simulink subsystem "S2"  (R2024b)
settings: Solver=VariableStepAuto  StartTime=0.0  StopTime=10.0  RelTol=1e-3
undefined symbols (not defined in the file): C, CC, DPL1ph, h, Half, Ll, nb_cell, numberOfCell, P_AC, Rdc, ResistanceM, Roff, Ron, Rt4, SampleTime, simetran, Ts, Zm
libraries: fl_lib x39, nesl_utility x33, ee_lib x20, simulink x6
(part 2 of 2)

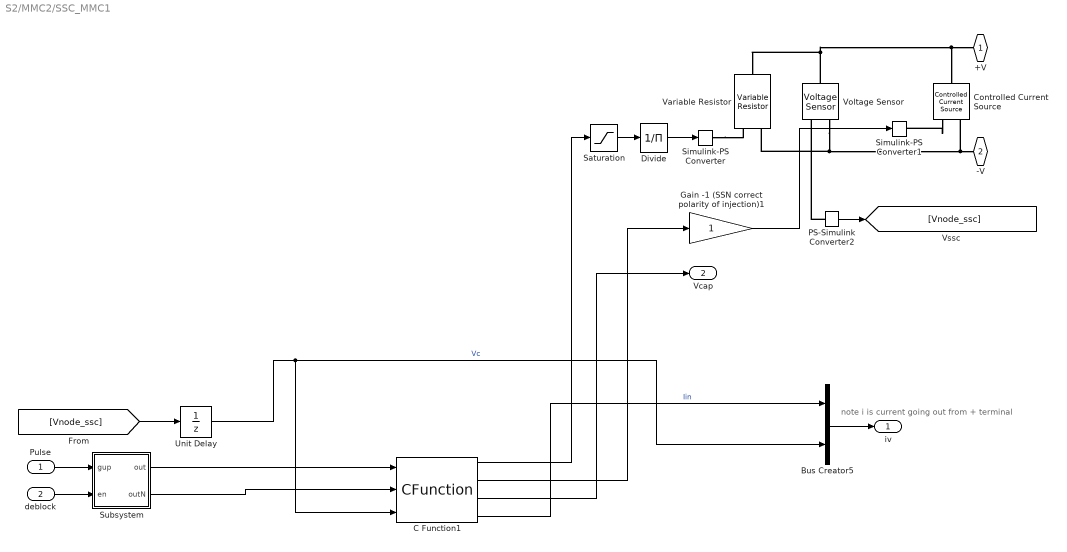
== system S2/MMC2/SSC_MMC1 ==
  note: note i is current going out from + terminal
  Pulse : Inport
  deblock : Inport  Port=2
  Bus Creator5 : BusCreator  Inputs=2
  C Function1 : CFunction  OutputCode=|  StartCode=state = initialValue;  InitializeConditionsCode=|  CodegenOutputCode=|  CodegenStartCode=state = initialValue;  CodegenInitializeConditionsCode=|  SampleTime=SampleTime  CustomCodeSettingLocation=ModelConfigurationParameters  initialValue=0  Ad=Ad  Bd2=Bd2  C=C  nbc=nbc  Z=Z  SampleTime=-1
      OutputCode=|
      | {
      | 
      | int ssx;
      | double Vcapasum, Ymmc, Zmmc, Vhist, Vterm;
      | double I;
      | 
      | Vcapasum=0;
      | I=(Vnodal- state_keep[0])* state_keep[1];  
      | 
      |     for (int k=0;k<nbc;k++){ //  % scan of cells to complete state-space iteration
      |         Vcap[k]=x_keep[k]+Bd2keep[k]*I;
      |         if (*(g_lower+k)<0.5) Vcapasum+=Vcap[k]; // sum all non-shorted capacitor voltages
      |     }
      | 
      | 
      |     Vhist=0;  // reset Vhist
      |     Zmmc=0;  // reset
      |     Vterm=  Vnodal;
      | 
      | 
      |     // we calculate the cells conduction states from the gate values.
      |     for (int k=0;k<nbc;k++){
      |         // ss=2-> lower IGBT/diode ON
      |         // ss=1-> upper IGBT/diode ON  //attention!!!!
      |         // ss=0-> hi-Z
      |         ssx=(int)gate[k];
      |         if (*(g_lower+k)>0.5) ssx=2;
      |         else if (*(g_upper+k)>0.5) ssx=1;
      |         else {
      |             if  (Vterm<0)  ssx=2;
      |             else if( Vterm>Vcapasum) ssx=1;
      |             else  ssx=0;
      |         }
      | 
      |         x_keep[k]=Ad[ssx]*Vcap[k];  //+Bd1[ssx]*I;    Bd1=0 avec backward Euler                                                          // note: with BE Bd1=0
      |         Vhist+=(C[ssx]*x_keep[k]);    //V_hist =V_hist + C(k)*state_tmp(k);  % compute Thevenin voltage
      | 
      |         Zmmc+=Z[ssx];  // Z = sum(C'.*Bd2 + D);  Y=inv(Z)
      | 
      |         Bd2keep[k]=Bd2[ssx];
      |         gate[k]=ssx;
      |         *(Vcap_out+k)=Vcap[k];
      |         }
      | 
      | 
      |     Ymmc=1/Zmmc;    // admittance= inverse of the sum of cell impedance
      |     Ihist=Vhist*Ymmc;  // history source
      | 
      |     state_keep[0]=Vhist;
      | 
      |     Y=Ymmc;
      | 
      |     state_keep[1]=Ymmc;
      | 
      |     Immc=0.0-I;
      | 
      | }
      InitializeConditionsCode=|
      | for (int i=0; i<nbc ;i++){
      |     x_keep[i]=0;
      |     Bd2keep[i]*0;
      |     Vc_state[i]=0;
      |     gate[i]=0;
      |     Vcap[i]=0;
      |     }
      |     
      |     state=0;
      |     state_keep[0]=0;
      |     state_keep[1]=0;
      CodegenOutputCode=|
      | {
      | 
      | int ssx;
      | double Vcapasum, Ymmc, Zmmc, Vhist, Vterm;
      | double I;
      | 
      | Vcapasum=0;
      | I=(Vnodal- state_keep[0])* state_keep[1];  
      | 
      |     for (int k=0;k<nbc;k++){ //  % scan of cells to complete state-space iteration
      |         Vcap[k]=x_keep[k]+Bd2keep[k]*I;
      |         if (*(g_lower+k)<0.5) Vcapasum+=Vcap[k]; // sum all non-shorted capacitor voltages
      |     }
      | 
      | 
      |     Vhist=0;  // reset Vhist
      |     Zmmc=0;  // reset
      |     Vterm=  Vnodal;
      | 
      | 
      |     // we calculate the cells conduction states from the gate values.
      |     for (int k=0;k<nbc;k++){
      |         // ss=2-> lower IGBT/diode ON
      |         // ss=1-> upper IGBT/diode ON  //attention!!!!
      |         // ss=0-> hi-Z
      |         ssx=(int)gate[k];
      |         if (*(g_lower+k)>0.5) ssx=2;
      |         else if (*(g_upper+k)>0.5) ssx=1;
      |         else {
      |             if  (Vterm<0)  ssx=2;
      |             else if( Vterm>Vcapasum) ssx=1;
      |             else  ssx=0;
      |         }
      | 
      |         x_keep[k]=Ad[ssx]*Vcap[k];  //+Bd1[ssx]*I;    Bd1=0 avec backward Euler                                                          // note: with BE Bd1=0
      |         Vhist+=(C[ssx]*x_keep[k]);    //V_hist =V_hist + C(k)*state_tmp(k);  % compute Thevenin voltage
      | 
      |         Zmmc+=Z[ssx];  // Z = sum(C'.*Bd2 + D);  Y=inv(Z)
      | 
      |         Bd2keep[k]=Bd2[ssx];
      |         gate[k]=ssx;
      |         *(Vcap_out+k)=Vcap[k];
      |         }
      | 
      | 
      |     Ymmc=1/Zmmc;    // admittance= inverse of the sum of cell impedance
      |     Ihist=Vhist*Ymmc;  // history source
      | 
      |     state_keep[0]=Vhist;
      | 
      |     Y=Ymmc;
      | 
      |     state_keep[1]=Ymmc;
      | 
      |     Immc=0.0-I;
      | 
      | }
      CodegenInitializeConditionsCode=|
      | for (int i=0; i<nbc ;i++){
      |     x_keep[i]=0;
      |     Bd2keep[i]*0;
      |     Vc_state[i]=0;
      |     gate[i]=0;
      |     Vcap[i]=0;
      |     }
      |     
      |     state=0;
      |     state_keep[0]=0;
      |     state_keep[1]=0;
  Controlled Current Source : fl_lib/Electrical/Electrical Sources/Controlled Current Source
  Divide : Product  Inputs=/
  Gain -1 (SSN correct polarity of injection)1 : Gain
  PS-Simulink Converter2 : nesl_utility/PS-Simulink Converter  PhysicalDomain=network_engine_domain  SubClassName=ps_output  LeftPortType=input  RightPortType=output  PseudoPeriodic=off  Frequencies=[]  VectorFormat=inherit  Unit=inherit  AffineConversion=off
  Saturation : Saturate  UpperLimit=1e9  LowerLimit=0
  Simulink-PS Converter : nesl_utility/Simulink-PS Converter  PhysicalDomain=network_engine_domain  SubClassName=ps_input  LeftPortType=input  RightPortType=output  PseudoPeriodic=off  Frequencies=[]  NoiseDistribution=none  NoiseParameters=[]  Unit=1  AffineConversion=off  FilteringAndDerivatives=provide  SimscapeFilterOrder=1  InputFilterTimeConstant=0.001  UdotUserProvided=0
  Simulink-PS Converter1 : nesl_utility/Simulink-PS Converter  PhysicalDomain=network_engine_domain  SubClassName=ps_input  LeftPortType=input  RightPortType=output  PseudoPeriodic=off  Frequencies=[]  NoiseDistribution=none  NoiseParameters=[]  Unit=1  AffineConversion=off  FilteringAndDerivatives=provide  SimscapeFilterOrder=1  InputFilterTimeConstant=0.001  UdotUserProvided=0
  Subsystem : Subsystem  mask(MMC pulsing){nbc=nbc}
      mask prompts: nbc "Number of Cells"
      mask init:
      | igbtorder=[];
      | for i=1:nbc
      |     igbtorder=[igbtorder i i+nbc];
      | end
      | igbtorder;
  Unit Delay : UnitDelay  SampleTime=Ts  HasFrameUpgradeWarning=on
  Variable Resistor : fl_lib/Electrical/Electrical Elements/Variable Resistor  Rmin=1e-8 Ohm  thermalEnable=false  thermal_mass=1 J/K  i_specify=off  i_priority=None  i=0 A  i_nominal_specify=off  i_nominal_value=1  i_nominal_unit=A  v_specify=off  v_priority=None  v=0 V  v_nominal_specify=off  v_nominal_value=1  v_nominal_unit=V  T_specify=off  T_priority=None  T=300 K  T_nominal_specify=off  T_nominal_value=1  T_nominal_unit=K
  Voltage Sensor : fl_lib/Electrical/Electrical Sensors/Voltage Sensor
  +V : PMIOPort  Side=Left
  -V : PMIOPort  Port=2  Side=Left
  iv : Outport  VectorParamsAs1DForOutWhenUnconnected=off
  Vcap : Outport  Port=2  VectorParamsAs1DForOutWhenUnconnected=off
  wires:
  C Function1/4 -> Bus Creator5/1  "Iin"
  C Function1/3 -> Vcap/1
  C Function1/2 -> Gain -1 (SSN correct polarity of injection)1/1
  C Function1/1 -> Saturation/1
  Unit Delay/1 -> Bus Creator5/2, C Function1/3  "Vc"
  Bus Creator5/1 -> iv/1
  Subsystem/1(out) -> C Function1/1
  Pulse/1 -> Subsystem/1(gup)
  Subsystem/2(outN) -> C Function1/2
  deblock/1 -> Subsystem/2(en)
  PS-Simulink Converter2/1 -> [Vnode_ssc]
  [Vnode_ssc] -> Unit Delay/1
  Gain -1 (SSN correct polarity of injection)1/1 -> Simulink-PS Converter1/1
  Divide/1 -> Simulink-PS Converter/1
  Saturation/1 -> Divide/1
  connections:
  Simulink-PS Converter/RConn1 -- Variable Resistor/LConn1
  Voltage Sensor/RConn2 -- Controlled Current Source/RConn2 -- -V/RConn1 -- Variable Resistor/LConn2
  Voltage Sensor/LConn1 -- Controlled Current Source/LConn1 -- +V/RConn1 -- Variable Resistor/RConn1
  PS-Simulink Converter2/LConn1 -- Voltage Sensor/RConn1
  Controlled Current Source/RConn1 -- Simulink-PS Converter1/RConn1

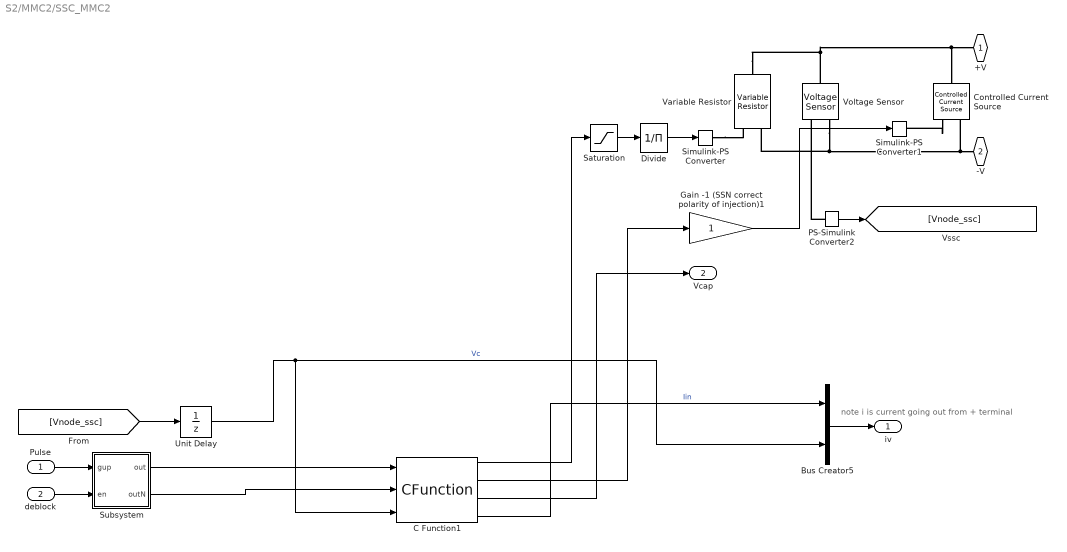
== system S2/MMC2/SSC_MMC2 ==
  note: note i is current going out from + terminal
  Pulse : Inport
  deblock : Inport  Port=2
  Bus Creator5 : BusCreator  Inputs=2
  C Function1 : CFunction  OutputCode=|  StartCode=state = initialValue;  InitializeConditionsCode=|  CodegenOutputCode=|  CodegenStartCode=state = initialValue;  CodegenInitializeConditionsCode=|  SampleTime=SampleTime  CustomCodeSettingLocation=ModelConfigurationParameters  initialValue=0  Ad=Ad  Bd2=Bd2  C=C  nbc=nbc  Z=Z  SampleTime=-1
      OutputCode=|
      | {
      | 
      | int ssx;
      | double Vcapasum, Ymmc, Zmmc, Vhist, Vterm;
      | double I;
      | 
      | Vcapasum=0;
      | I=(Vnodal- state_keep[0])* state_keep[1];  
      | 
      |     for (int k=0;k<nbc;k++){ //  % scan of cells to complete state-space iteration
      |         Vcap[k]=x_keep[k]+Bd2keep[k]*I;
      |         if (*(g_lower+k)<0.5) Vcapasum+=Vcap[k]; // sum all non-shorted capacitor voltages
      |     }
      | 
      | 
      |     Vhist=0;  // reset Vhist
      |     Zmmc=0;  // reset
      |     Vterm=  Vnodal;
      | 
      | 
      |     // we calculate the cells conduction states from the gate values.
      |     for (int k=0;k<nbc;k++){
      |         // ss=2-> lower IGBT/diode ON
      |         // ss=1-> upper IGBT/diode ON  //attention!!!!
      |         // ss=0-> hi-Z
      |         ssx=(int)gate[k];
      |         if (*(g_lower+k)>0.5) ssx=2;
      |         else if (*(g_upper+k)>0.5) ssx=1;
      |         else {
      |             if  (Vterm<0)  ssx=2;
      |             else if( Vterm>Vcapasum) ssx=1;
      |             else  ssx=0;
      |         }
      | 
      |         x_keep[k]=Ad[ssx]*Vcap[k];  //+Bd1[ssx]*I;    Bd1=0 avec backward Euler                                                          // note: with BE Bd1=0
      |         Vhist+=(C[ssx]*x_keep[k]);    //V_hist =V_hist + C(k)*state_tmp(k);  % compute Thevenin voltage
      | 
      |         Zmmc+=Z[ssx];  // Z = sum(C'.*Bd2 + D);  Y=inv(Z)
      | 
      |         Bd2keep[k]=Bd2[ssx];
      |         gate[k]=ssx;
      |         *(Vcap_out+k)=Vcap[k];
      |         }
      | 
      | 
      |     Ymmc=1/Zmmc;    // admittance= inverse of the sum of cell impedance
      |     Ihist=Vhist*Ymmc;  // history source
      | 
      |     state_keep[0]=Vhist;
      | 
      |     Y=Ymmc;
      | 
      |     state_keep[1]=Ymmc;
      | 
      |     Immc=0.0-I;
      | 
      | }
      InitializeConditionsCode=|
      | for (int i=0; i<nbc ;i++){
      |     x_keep[i]=0;
      |     Bd2keep[i]*0;
      |     Vc_state[i]=0;
      |     gate[i]=0;
      |     Vcap[i]=0;
      |     }
      |     
      |     state=0;
      |     state_keep[0]=0;
      |     state_keep[1]=0;
      CodegenOutputCode=|
      | {
      | 
      | int ssx;
      | double Vcapasum, Ymmc, Zmmc, Vhist, Vterm;
      | double I;
      | 
      | Vcapasum=0;
      | I=(Vnodal- state_keep[0])* state_keep[1];  
      | 
      |     for (int k=0;k<nbc;k++){ //  % scan of cells to complete state-space iteration
      |         Vcap[k]=x_keep[k]+Bd2keep[k]*I;
      |         if (*(g_lower+k)<0.5) Vcapasum+=Vcap[k]; // sum all non-shorted capacitor voltages
      |     }
      | 
      | 
      |     Vhist=0;  // reset Vhist
      |     Zmmc=0;  // reset
      |     Vterm=  Vnodal;
      | 
      | 
      |     // we calculate the cells conduction states from the gate values.
      |     for (int k=0;k<nbc;k++){
      |         // ss=2-> lower IGBT/diode ON
      |         // ss=1-> upper IGBT/diode ON  //attention!!!!
      |         // ss=0-> hi-Z
      |         ssx=(int)gate[k];
      |         if (*(g_lower+k)>0.5) ssx=2;
      |         else if (*(g_upper+k)>0.5) ssx=1;
      |         else {
      |             if  (Vterm<0)  ssx=2;
      |             else if( Vterm>Vcapasum) ssx=1;
      |             else  ssx=0;
      |         }
      | 
      |         x_keep[k]=Ad[ssx]*Vcap[k];  //+Bd1[ssx]*I;    Bd1=0 avec backward Euler                                                          // note: with BE Bd1=0
      |         Vhist+=(C[ssx]*x_keep[k]);    //V_hist =V_hist + C(k)*state_tmp(k);  % compute Thevenin voltage
      | 
      |         Zmmc+=Z[ssx];  // Z = sum(C'.*Bd2 + D);  Y=inv(Z)
      | 
      |         Bd2keep[k]=Bd2[ssx];
      |         gate[k]=ssx;
      |         *(Vcap_out+k)=Vcap[k];
      |         }
      | 
      | 
      |     Ymmc=1/Zmmc;    // admittance= inverse of the sum of cell impedance
      |     Ihist=Vhist*Ymmc;  // history source
      | 
      |     state_keep[0]=Vhist;
      | 
      |     Y=Ymmc;
      | 
      |     state_keep[1]=Ymmc;
      | 
      |     Immc=0.0-I;
      | 
      | }
      CodegenInitializeConditionsCode=|
      | for (int i=0; i<nbc ;i++){
      |     x_keep[i]=0;
      |     Bd2keep[i]*0;
      |     Vc_state[i]=0;
      |     gate[i]=0;
      |     Vcap[i]=0;
      |     }
      |     
      |     state=0;
      |     state_keep[0]=0;
      |     state_keep[1]=0;
  Controlled Current Source : fl_lib/Electrical/Electrical Sources/Controlled Current Source
  Divide : Product  Inputs=/
  Gain -1 (SSN correct polarity of injection)1 : Gain
  PS-Simulink Converter2 : nesl_utility/PS-Simulink Converter  PhysicalDomain=network_engine_domain  SubClassName=ps_output  LeftPortType=input  RightPortType=output  PseudoPeriodic=off  Frequencies=[]  VectorFormat=inherit  Unit=inherit  AffineConversion=off
  Saturation : Saturate  UpperLimit=1e9  LowerLimit=0
  Simulink-PS Converter : nesl_utility/Simulink-PS Converter  PhysicalDomain=network_engine_domain  SubClassName=ps_input  LeftPortType=input  RightPortType=output  PseudoPeriodic=off  Frequencies=[]  NoiseDistribution=none  NoiseParameters=[]  Unit=1  AffineConversion=off  FilteringAndDerivatives=provide  SimscapeFilterOrder=1  InputFilterTimeConstant=0.001  UdotUserProvided=0
  Simulink-PS Converter1 : nesl_utility/Simulink-PS Converter  PhysicalDomain=network_engine_domain  SubClassName=ps_input  LeftPortType=input  RightPortType=output  PseudoPeriodic=off  Frequencies=[]  NoiseDistribution=none  NoiseParameters=[]  Unit=1  AffineConversion=off  FilteringAndDerivatives=provide  SimscapeFilterOrder=1  InputFilterTimeConstant=0.001  UdotUserProvided=0
  Subsystem : Subsystem  mask(MMC pulsing){nbc=nbc}
      mask prompts: nbc "Number of Cells"
      mask init:
      | igbtorder=[];
      | for i=1:nbc
      |     igbtorder=[igbtorder i i+nbc];
      | end
      | igbtorder;
  Unit Delay : UnitDelay  SampleTime=Ts  HasFrameUpgradeWarning=on
  Variable Resistor : fl_lib/Electrical/Electrical Elements/Variable Resistor  Rmin=1e-8 Ohm  thermalEnable=false  thermal_mass=1 J/K  i_specify=off  i_priority=None  i=0 A  i_nominal_specify=off  i_nominal_value=1  i_nominal_unit=A  v_specify=off  v_priority=None  v=0 V  v_nominal_specify=off  v_nominal_value=1  v_nominal_unit=V  T_specify=off  T_priority=None  T=300 K  T_nominal_specify=off  T_nominal_value=1  T_nominal_unit=K
  Voltage Sensor : fl_lib/Electrical/Electrical Sensors/Voltage Sensor
  +V : PMIOPort  Side=Left
  -V : PMIOPort  Port=2  Side=Left
  iv : Outport  VectorParamsAs1DForOutWhenUnconnected=off
  Vcap : Outport  Port=2  VectorParamsAs1DForOutWhenUnconnected=off
  wires:
  Saturation/1 -> Divide/1
  Divide/1 -> Simulink-PS Converter/1
  Gain -1 (SSN correct polarity of injection)1/1 -> Simulink-PS Converter1/1
  [Vnode_ssc] -> Unit Delay/1
  PS-Simulink Converter2/1 -> [Vnode_ssc]
  deblock/1 -> Subsystem/2(en)
  Subsystem/2(outN) -> C Function1/2
  Pulse/1 -> Subsystem/1(gup)
  Subsystem/1(out) -> C Function1/1
  Bus Creator5/1 -> iv/1
  Unit Delay/1 -> C Function1/3, Bus Creator5/2  "Vc"
  C Function1/1 -> Saturation/1
  C Function1/2 -> Gain -1 (SSN correct polarity of injection)1/1
  C Function1/3 -> Vcap/1
  C Function1/4 -> Bus Creator5/1  "Iin"
  connections:
  Controlled Current Source/RConn1 -- Simulink-PS Converter1/RConn1
  PS-Simulink Converter2/LConn1 -- Voltage Sensor/RConn1
  Variable Resistor/RConn1 -- +V/RConn1 -- Controlled Current Source/LConn1 -- Voltage Sensor/LConn1
  Variable Resistor/LConn2 -- -V/RConn1 -- Controlled Current Source/RConn2 -- Voltage Sensor/RConn2
  Simulink-PS Converter/RConn1 -- Variable Resistor/LConn1

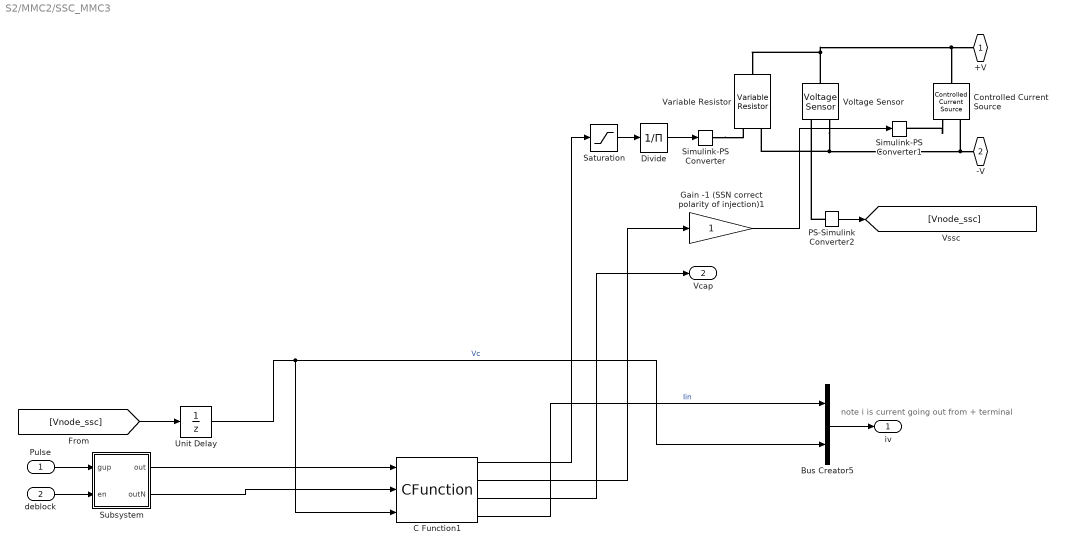
== system S2/MMC2/SSC_MMC3 ==
  note: note i is current going out from + terminal
  Pulse : Inport
  deblock : Inport  Port=2
  Bus Creator5 : BusCreator  Inputs=2
  C Function1 : CFunction  OutputCode=|  StartCode=state = initialValue;  InitializeConditionsCode=|  CodegenOutputCode=|  CodegenStartCode=state = initialValue;  CodegenInitializeConditionsCode=|  SampleTime=SampleTime  CustomCodeSettingLocation=ModelConfigurationParameters  initialValue=0  Ad=Ad  Bd2=Bd2  C=C  nbc=nbc  Z=Z  SampleTime=-1
      OutputCode=|
      | {
      | 
      | int ssx;
      | double Vcapasum, Ymmc, Zmmc, Vhist, Vterm;
      | double I;
      | 
      | Vcapasum=0;
      | I=(Vnodal- state_keep[0])* state_keep[1];  
      | 
      |     for (int k=0;k<nbc;k++){ //  % scan of cells to complete state-space iteration
      |         Vcap[k]=x_keep[k]+Bd2keep[k]*I;
      |         if (*(g_lower+k)<0.5) Vcapasum+=Vcap[k]; // sum all non-shorted capacitor voltages
      |     }
      | 
      | 
      |     Vhist=0;  // reset Vhist
      |     Zmmc=0;  // reset
      |     Vterm=  Vnodal;
      | 
      | 
      |     // we calculate the cells conduction states from the gate values.
      |     for (int k=0;k<nbc;k++){
      |         // ss=2-> lower IGBT/diode ON
      |         // ss=1-> upper IGBT/diode ON  //attention!!!!
      |         // ss=0-> hi-Z
      |         ssx=(int)gate[k];
      |         if (*(g_lower+k)>0.5) ssx=2;
      |         else if (*(g_upper+k)>0.5) ssx=1;
      |         else {
      |             if  (Vterm<0)  ssx=2;
      |             else if( Vterm>Vcapasum) ssx=1;
      |             else  ssx=0;
      |         }
      | 
      |         x_keep[k]=Ad[ssx]*Vcap[k];  //+Bd1[ssx]*I;    Bd1=0 avec backward Euler                                                          // note: with BE Bd1=0
      |         Vhist+=(C[ssx]*x_keep[k]);    //V_hist =V_hist + C(k)*state_tmp(k);  % compute Thevenin voltage
      | 
      |         Zmmc+=Z[ssx];  // Z = sum(C'.*Bd2 + D);  Y=inv(Z)
      | 
      |         Bd2keep[k]=Bd2[ssx];
      |         gate[k]=ssx;
      |         *(Vcap_out+k)=Vcap[k];
      |         }
      | 
      | 
      |     Ymmc=1/Zmmc;    // admittance= inverse of the sum of cell impedance
      |     Ihist=Vhist*Ymmc;  // history source
      | 
      |     state_keep[0]=Vhist;
      | 
      |     Y=Ymmc;
      | 
      |     state_keep[1]=Ymmc;
      | 
      |     Immc=0.0-I;
      | 
      | }
      InitializeConditionsCode=|
      | for (int i=0; i<nbc ;i++){
      |     x_keep[i]=0;
      |     Bd2keep[i]*0;
      |     Vc_state[i]=0;
      |     gate[i]=0;
      |     Vcap[i]=0;
      |     }
      |     
      |     state=0;
      |     state_keep[0]=0;
      |     state_keep[1]=0;
      CodegenOutputCode=|
      | {
      | 
      | int ssx;
      | double Vcapasum, Ymmc, Zmmc, Vhist, Vterm;
      | double I;
      | 
      | Vcapasum=0;
      | I=(Vnodal- state_keep[0])* state_keep[1];  
      | 
      |     for (int k=0;k<nbc;k++){ //  % scan of cells to complete state-space iteration
      |         Vcap[k]=x_keep[k]+Bd2keep[k]*I;
      |         if (*(g_lower+k)<0.5) Vcapasum+=Vcap[k]; // sum all non-shorted capacitor voltages
      |     }
      | 
      | 
      |     Vhist=0;  // reset Vhist
      |     Zmmc=0;  // reset
      |     Vterm=  Vnodal;
      | 
      | 
      |     // we calculate the cells conduction states from the gate values.
      |     for (int k=0;k<nbc;k++){
      |         // ss=2-> lower IGBT/diode ON
      |         // ss=1-> upper IGBT/diode ON  //attention!!!!
      |         // ss=0-> hi-Z
      |         ssx=(int)gate[k];
      |         if (*(g_lower+k)>0.5) ssx=2;
      |         else if (*(g_upper+k)>0.5) ssx=1;
      |         else {
      |             if  (Vterm<0)  ssx=2;
      |             else if( Vterm>Vcapasum) ssx=1;
      |             else  ssx=0;
      |         }
      | 
      |         x_keep[k]=Ad[ssx]*Vcap[k];  //+Bd1[ssx]*I;    Bd1=0 avec backward Euler                                                          // note: with BE Bd1=0
      |         Vhist+=(C[ssx]*x_keep[k]);    //V_hist =V_hist + C(k)*state_tmp(k);  % compute Thevenin voltage
      | 
      |         Zmmc+=Z[ssx];  // Z = sum(C'.*Bd2 + D);  Y=inv(Z)
      | 
      |         Bd2keep[k]=Bd2[ssx];
      |         gate[k]=ssx;
      |         *(Vcap_out+k)=Vcap[k];
      |         }
      | 
      | 
      |     Ymmc=1/Zmmc;    // admittance= inverse of the sum of cell impedance
      |     Ihist=Vhist*Ymmc;  // history source
      | 
      |     state_keep[0]=Vhist;
      | 
      |     Y=Ymmc;
      | 
      |     state_keep[1]=Ymmc;
      | 
      |     Immc=0.0-I;
      | 
      | }
      CodegenInitializeConditionsCode=|
      | for (int i=0; i<nbc ;i++){
      |     x_keep[i]=0;
      |     Bd2keep[i]*0;
      |     Vc_state[i]=0;
      |     gate[i]=0;
      |     Vcap[i]=0;
      |     }
      |     
      |     state=0;
      |     state_keep[0]=0;
      |     state_keep[1]=0;
  Controlled Current Source : fl_lib/Electrical/Electrical Sources/Controlled Current Source
  Divide : Product  Inputs=/
  Gain -1 (SSN correct polarity of injection)1 : Gain
  PS-Simulink Converter2 : nesl_utility/PS-Simulink Converter  PhysicalDomain=network_engine_domain  SubClassName=ps_output  LeftPortType=input  RightPortType=output  PseudoPeriodic=off  Frequencies=[]  VectorFormat=inherit  Unit=inherit  AffineConversion=off
  Saturation : Saturate  UpperLimit=1e9  LowerLimit=0
  Simulink-PS Converter : nesl_utility/Simulink-PS Converter  PhysicalDomain=network_engine_domain  SubClassName=ps_input  LeftPortType=input  RightPortType=output  PseudoPeriodic=off  Frequencies=[]  NoiseDistribution=none  NoiseParameters=[]  Unit=1  AffineConversion=off  FilteringAndDerivatives=provide  SimscapeFilterOrder=1  InputFilterTimeConstant=0.001  UdotUserProvided=0
  Simulink-PS Converter1 : nesl_utility/Simulink-PS Converter  PhysicalDomain=network_engine_domain  SubClassName=ps_input  LeftPortType=input  RightPortType=output  PseudoPeriodic=off  Frequencies=[]  NoiseDistribution=none  NoiseParameters=[]  Unit=1  AffineConversion=off  FilteringAndDerivatives=provide  SimscapeFilterOrder=1  InputFilterTimeConstant=0.001  UdotUserProvided=0
  Subsystem : Subsystem  mask(MMC pulsing){nbc=nbc}
      mask prompts: nbc "Number of Cells"
      mask init:
      | igbtorder=[];
      | for i=1:nbc
      |     igbtorder=[igbtorder i i+nbc];
      | end
      | igbtorder;
  Unit Delay : UnitDelay  SampleTime=Ts  HasFrameUpgradeWarning=on
  Variable Resistor : fl_lib/Electrical/Electrical Elements/Variable Resistor  Rmin=1e-8 Ohm  thermalEnable=false  thermal_mass=1 J/K  i_specify=off  i_priority=None  i=0 A  i_nominal_specify=off  i_nominal_value=1  i_nominal_unit=A  v_specify=off  v_priority=None  v=0 V  v_nominal_specify=off  v_nominal_value=1  v_nominal_unit=V  T_specify=off  T_priority=None  T=300 K  T_nominal_specify=off  T_nominal_value=1  T_nominal_unit=K
  Voltage Sensor : fl_lib/Electrical/Electrical Sensors/Voltage Sensor
  +V : PMIOPort  Side=Left
  -V : PMIOPort  Port=2  Side=Left
  iv : Outport  VectorParamsAs1DForOutWhenUnconnected=off
  Vcap : Outport  Port=2  VectorParamsAs1DForOutWhenUnconnected=off
  wires:
  C Function1/4 -> Bus Creator5/1  "Iin"
  C Function1/3 -> Vcap/1
  C Function1/2 -> Gain -1 (SSN correct polarity of injection)1/1
  C Function1/1 -> Saturation/1
  Unit Delay/1 -> Bus Creator5/2, C Function1/3  "Vc"
  Bus Creator5/1 -> iv/1
  Subsystem/1(out) -> C Function1/1
  Pulse/1 -> Subsystem/1(gup)
  Subsystem/2(outN) -> C Function1/2
  deblock/1 -> Subsystem/2(en)
  PS-Simulink Converter2/1 -> [Vnode_ssc]
  [Vnode_ssc] -> Unit Delay/1
  Gain -1 (SSN correct polarity of injection)1/1 -> Simulink-PS Converter1/1
  Divide/1 -> Simulink-PS Converter/1
  Saturation/1 -> Divide/1
  connections:
  Simulink-PS Converter/RConn1 -- Variable Resistor/LConn1
  Voltage Sensor/RConn2 -- Controlled Current Source/RConn2 -- -V/RConn1 -- Variable Resistor/LConn2
  Voltage Sensor/LConn1 -- Controlled Current Source/LConn1 -- +V/RConn1 -- Variable Resistor/RConn1
  PS-Simulink Converter2/LConn1 -- Voltage Sensor/RConn1
  Controlled Current Source/RConn1 -- Simulink-PS Converter1/RConn1

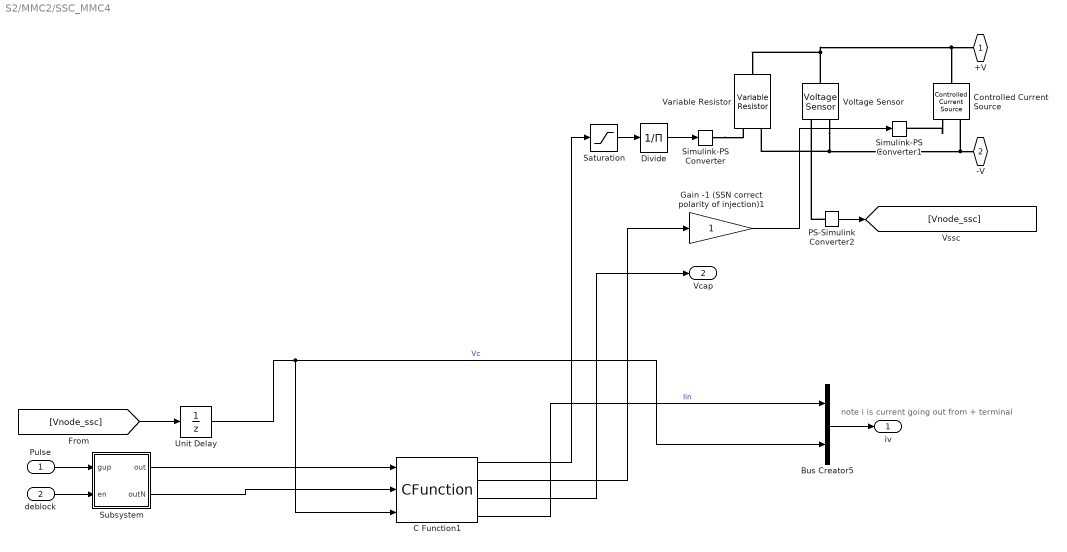
== system S2/MMC2/SSC_MMC4 ==
  note: note i is current going out from + terminal
  Pulse : Inport
  deblock : Inport  Port=2
  Bus Creator5 : BusCreator  Inputs=2
  C Function1 : CFunction  OutputCode=|  StartCode=state = initialValue;  InitializeConditionsCode=|  CodegenOutputCode=|  CodegenStartCode=state = initialValue;  CodegenInitializeConditionsCode=|  SampleTime=SampleTime  CustomCodeSettingLocation=ModelConfigurationParameters  initialValue=0  Ad=Ad  Bd2=Bd2  C=C  nbc=nbc  Z=Z  SampleTime=-1
      OutputCode=|
      | {
      | 
      | int ssx;
      | double Vcapasum, Ymmc, Zmmc, Vhist, Vterm;
      | double I;
      | 
      | Vcapasum=0;
      | I=(Vnodal- state_keep[0])* state_keep[1];  
      | 
      |     for (int k=0;k<nbc;k++){ //  % scan of cells to complete state-space iteration
      |         Vcap[k]=x_keep[k]+Bd2keep[k]*I;
      |         if (*(g_lower+k)<0.5) Vcapasum+=Vcap[k]; // sum all non-shorted capacitor voltages
      |     }
      | 
      | 
      |     Vhist=0;  // reset Vhist
      |     Zmmc=0;  // reset
      |     Vterm=  Vnodal;
      | 
      | 
      |     // we calculate the cells conduction states from the gate values.
      |     for (int k=0;k<nbc;k++){
      |         // ss=2-> lower IGBT/diode ON
      |         // ss=1-> upper IGBT/diode ON  //attention!!!!
      |         // ss=0-> hi-Z
      |         ssx=(int)gate[k];
      |         if (*(g_lower+k)>0.5) ssx=2;
      |         else if (*(g_upper+k)>0.5) ssx=1;
      |         else {
      |             if  (Vterm<0)  ssx=2;
      |             else if( Vterm>Vcapasum) ssx=1;
      |             else  ssx=0;
      |         }
      | 
      |         x_keep[k]=Ad[ssx]*Vcap[k];  //+Bd1[ssx]*I;    Bd1=0 avec backward Euler                                                          // note: with BE Bd1=0
      |         Vhist+=(C[ssx]*x_keep[k]);    //V_hist =V_hist + C(k)*state_tmp(k);  % compute Thevenin voltage
      | 
      |         Zmmc+=Z[ssx];  // Z = sum(C'.*Bd2 + D);  Y=inv(Z)
      | 
      |         Bd2keep[k]=Bd2[ssx];
      |         gate[k]=ssx;
      |         *(Vcap_out+k)=Vcap[k];
      |         }
      | 
      | 
      |     Ymmc=1/Zmmc;    // admittance= inverse of the sum of cell impedance
      |     Ihist=Vhist*Ymmc;  // history source
      | 
      |     state_keep[0]=Vhist;
      | 
      |     Y=Ymmc;
      | 
      |     state_keep[1]=Ymmc;
      | 
      |     Immc=0.0-I;
      | 
      | }
      InitializeConditionsCode=|
      | for (int i=0; i<nbc ;i++){
      |     x_keep[i]=0;
      |     Bd2keep[i]*0;
      |     Vc_state[i]=0;
      |     gate[i]=0;
      |     Vcap[i]=0;
      |     }
      |     
      |     state=0;
      |     state_keep[0]=0;
      |     state_keep[1]=0;
      CodegenOutputCode=|
      | {
      | 
      | int ssx;
      | double Vcapasum, Ymmc, Zmmc, Vhist, Vterm;
      | double I;
      | 
      | Vcapasum=0;
      | I=(Vnodal- state_keep[0])* state_keep[1];  
      | 
      |     for (int k=0;k<nbc;k++){ //  % scan of cells to complete state-space iteration
      |         Vcap[k]=x_keep[k]+Bd2keep[k]*I;
      |         if (*(g_lower+k)<0.5) Vcapasum+=Vcap[k]; // sum all non-shorted capacitor voltages
      |     }
      | 
      | 
      |     Vhist=0;  // reset Vhist
      |     Zmmc=0;  // reset
      |     Vterm=  Vnodal;
      | 
      | 
      |     // we calculate the cells conduction states from the gate values.
      |     for (int k=0;k<nbc;k++){
      |         // ss=2-> lower IGBT/diode ON
      |         // ss=1-> upper IGBT/diode ON  //attention!!!!
      |         // ss=0-> hi-Z
      |         ssx=(int)gate[k];
      |         if (*(g_lower+k)>0.5) ssx=2;
      |         else if (*(g_upper+k)>0.5) ssx=1;
      |         else {
      |             if  (Vterm<0)  ssx=2;
      |             else if( Vterm>Vcapasum) ssx=1;
      |             else  ssx=0;
      |         }
      | 
      |         x_keep[k]=Ad[ssx]*Vcap[k];  //+Bd1[ssx]*I;    Bd1=0 avec backward Euler                                                          // note: with BE Bd1=0
      |         Vhist+=(C[ssx]*x_keep[k]);    //V_hist =V_hist + C(k)*state_tmp(k);  % compute Thevenin voltage
      | 
      |         Zmmc+=Z[ssx];  // Z = sum(C'.*Bd2 + D);  Y=inv(Z)
      | 
      |         Bd2keep[k]=Bd2[ssx];
      |         gate[k]=ssx;
      |         *(Vcap_out+k)=Vcap[k];
      |         }
      | 
      | 
      |     Ymmc=1/Zmmc;    // admittance= inverse of the sum of cell impedance
      |     Ihist=Vhist*Ymmc;  // history source
      | 
      |     state_keep[0]=Vhist;
      | 
      |     Y=Ymmc;
      | 
      |     state_keep[1]=Ymmc;
      | 
      |     Immc=0.0-I;
      | 
      | }
      CodegenInitializeConditionsCode=|
      | for (int i=0; i<nbc ;i++){
      |     x_keep[i]=0;
      |     Bd2keep[i]*0;
      |     Vc_state[i]=0;
      |     gate[i]=0;
      |     Vcap[i]=0;
      |     }
      |     
      |     state=0;
      |     state_keep[0]=0;
      |     state_keep[1]=0;
  Controlled Current Source : fl_lib/Electrical/Electrical Sources/Controlled Current Source
  Divide : Product  Inputs=/
  Gain -1 (SSN correct polarity of injection)1 : Gain
  PS-Simulink Converter2 : nesl_utility/PS-Simulink Converter  PhysicalDomain=network_engine_domain  SubClassName=ps_output  LeftPortType=input  RightPortType=output  PseudoPeriodic=off  Frequencies=[]  VectorFormat=inherit  Unit=inherit  AffineConversion=off
  Saturation : Saturate  UpperLimit=1e9  LowerLimit=0
  Simulink-PS Converter : nesl_utility/Simulink-PS Converter  PhysicalDomain=network_engine_domain  SubClassName=ps_input  LeftPortType=input  RightPortType=output  PseudoPeriodic=off  Frequencies=[]  NoiseDistribution=none  NoiseParameters=[]  Unit=1  AffineConversion=off  FilteringAndDerivatives=provide  SimscapeFilterOrder=1  InputFilterTimeConstant=0.001  UdotUserProvided=0
  Simulink-PS Converter1 : nesl_utility/Simulink-PS Converter  PhysicalDomain=network_engine_domain  SubClassName=ps_input  LeftPortType=input  RightPortType=output  PseudoPeriodic=off  Frequencies=[]  NoiseDistribution=none  NoiseParameters=[]  Unit=1  AffineConversion=off  FilteringAndDerivatives=provide  SimscapeFilterOrder=1  InputFilterTimeConstant=0.001  UdotUserProvided=0
  Subsystem : Subsystem  mask(MMC pulsing){nbc=nbc}
      mask prompts: nbc "Number of Cells"
      mask init:
      | igbtorder=[];
      | for i=1:nbc
      |     igbtorder=[igbtorder i i+nbc];
      | end
      | igbtorder;
  Unit Delay : UnitDelay  SampleTime=Ts  HasFrameUpgradeWarning=on
  Variable Resistor : fl_lib/Electrical/Electrical Elements/Variable Resistor  Rmin=1e-8 Ohm  thermalEnable=false  thermal_mass=1 J/K  i_specify=off  i_priority=None  i=0 A  i_nominal_specify=off  i_nominal_value=1  i_nominal_unit=A  v_specify=off  v_priority=None  v=0 V  v_nominal_specify=off  v_nominal_value=1  v_nominal_unit=V  T_specify=off  T_priority=None  T=300 K  T_nominal_specify=off  T_nominal_value=1  T_nominal_unit=K
  Voltage Sensor : fl_lib/Electrical/Electrical Sensors/Voltage Sensor
  +V : PMIOPort  Side=Left
  -V : PMIOPort  Port=2  Side=Left
  iv : Outport  VectorParamsAs1DForOutWhenUnconnected=off
  Vcap : Outport  Port=2  VectorParamsAs1DForOutWhenUnconnected=off
  wires:
  C Function1/4 -> Bus Creator5/1  "Iin"
  C Function1/3 -> Vcap/1
  C Function1/2 -> Gain -1 (SSN correct polarity of injection)1/1
  C Function1/1 -> Saturation/1
  Unit Delay/1 -> Bus Creator5/2, C Function1/3  "Vc"
  Bus Creator5/1 -> iv/1
  Subsystem/1(out) -> C Function1/1
  Pulse/1 -> Subsystem/1(gup)
  Subsystem/2(outN) -> C Function1/2
  deblock/1 -> Subsystem/2(en)
  PS-Simulink Converter2/1 -> [Vnode_ssc]
  [Vnode_ssc] -> Unit Delay/1
  Gain -1 (SSN correct polarity of injection)1/1 -> Simulink-PS Converter1/1
  Divide/1 -> Simulink-PS Converter/1
  Saturation/1 -> Divide/1
  connections:
  Simulink-PS Converter/RConn1 -- Variable Resistor/LConn1
  Voltage Sensor/RConn2 -- Controlled Current Source/RConn2 -- -V/RConn1 -- Variable Resistor/LConn2
  Voltage Sensor/LConn1 -- Controlled Current Source/LConn1 -- +V/RConn1 -- Variable Resistor/RConn1
  PS-Simulink Converter2/LConn1 -- Voltage Sensor/RConn1
  Controlled Current Source/RConn1 -- Simulink-PS Converter1/RConn1

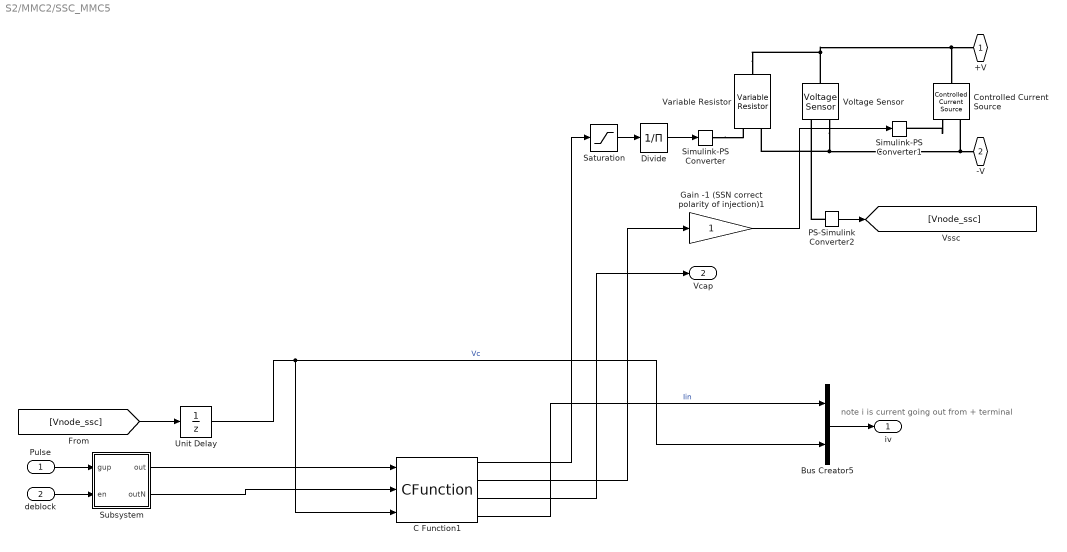
== system S2/MMC2/SSC_MMC5 ==
  note: note i is current going out from + terminal
  Pulse : Inport
  deblock : Inport  Port=2
  Bus Creator5 : BusCreator  Inputs=2
  C Function1 : CFunction  OutputCode=|  StartCode=state = initialValue;  InitializeConditionsCode=|  CodegenOutputCode=|  CodegenStartCode=state = initialValue;  CodegenInitializeConditionsCode=|  SampleTime=SampleTime  CustomCodeSettingLocation=ModelConfigurationParameters  initialValue=0  Ad=Ad  Bd2=Bd2  C=C  nbc=nbc  Z=Z  SampleTime=-1
      OutputCode=|
      | {
      | 
      | int ssx;
      | double Vcapasum, Ymmc, Zmmc, Vhist, Vterm;
      | double I;
      | 
      | Vcapasum=0;
      | I=(Vnodal- state_keep[0])* state_keep[1];  
      | 
      |     for (int k=0;k<nbc;k++){ //  % scan of cells to complete state-space iteration
      |         Vcap[k]=x_keep[k]+Bd2keep[k]*I;
      |         if (*(g_lower+k)<0.5) Vcapasum+=Vcap[k]; // sum all non-shorted capacitor voltages
      |     }
      | 
      | 
      |     Vhist=0;  // reset Vhist
      |     Zmmc=0;  // reset
      |     Vterm=  Vnodal;
      | 
      | 
      |     // we calculate the cells conduction states from the gate values.
      |     for (int k=0;k<nbc;k++){
      |         // ss=2-> lower IGBT/diode ON
      |         // ss=1-> upper IGBT/diode ON  //attention!!!!
      |         // ss=0-> hi-Z
      |         ssx=(int)gate[k];
      |         if (*(g_lower+k)>0.5) ssx=2;
      |         else if (*(g_upper+k)>0.5) ssx=1;
      |         else {
      |             if  (Vterm<0)  ssx=2;
      |             else if( Vterm>Vcapasum) ssx=1;
      |             else  ssx=0;
      |         }
      | 
      |         x_keep[k]=Ad[ssx]*Vcap[k];  //+Bd1[ssx]*I;    Bd1=0 avec backward Euler                                                          // note: with BE Bd1=0
      |         Vhist+=(C[ssx]*x_keep[k]);    //V_hist =V_hist + C(k)*state_tmp(k);  % compute Thevenin voltage
      | 
      |         Zmmc+=Z[ssx];  // Z = sum(C'.*Bd2 + D);  Y=inv(Z)
      | 
      |         Bd2keep[k]=Bd2[ssx];
      |         gate[k]=ssx;
      |         *(Vcap_out+k)=Vcap[k];
      |         }
      | 
      | 
      |     Ymmc=1/Zmmc;    // admittance= inverse of the sum of cell impedance
      |     Ihist=Vhist*Ymmc;  // history source
      | 
      |     state_keep[0]=Vhist;
      | 
      |     Y=Ymmc;
      | 
      |     state_keep[1]=Ymmc;
      | 
      |     Immc=0.0-I;
      | 
      | }
      InitializeConditionsCode=|
      | for (int i=0; i<nbc ;i++){
      |     x_keep[i]=0;
      |     Bd2keep[i]*0;
      |     Vc_state[i]=0;
      |     gate[i]=0;
      |     Vcap[i]=0;
      |     }
      |     
      |     state=0;
      |     state_keep[0]=0;
      |     state_keep[1]=0;
      CodegenOutputCode=|
      | {
      | 
      | int ssx;
      | double Vcapasum, Ymmc, Zmmc, Vhist, Vterm;
      | double I;
      | 
      | Vcapasum=0;
      | I=(Vnodal- state_keep[0])* state_keep[1];  
      | 
      |     for (int k=0;k<nbc;k++){ //  % scan of cells to complete state-space iteration
      |         Vcap[k]=x_keep[k]+Bd2keep[k]*I;
      |         if (*(g_lower+k)<0.5) Vcapasum+=Vcap[k]; // sum all non-shorted capacitor voltages
      |     }
      | 
      | 
      |     Vhist=0;  // reset Vhist
      |     Zmmc=0;  // reset
      |     Vterm=  Vnodal;
      | 
      | 
      |     // we calculate the cells conduction states from the gate values.
      |     for (int k=0;k<nbc;k++){
      |         // ss=2-> lower IGBT/diode ON
      |         // ss=1-> upper IGBT/diode ON  //attention!!!!
      |         // ss=0-> hi-Z
      |         ssx=(int)gate[k];
      |         if (*(g_lower+k)>0.5) ssx=2;
      |         else if (*(g_upper+k)>0.5) ssx=1;
      |         else {
      |             if  (Vterm<0)  ssx=2;
      |             else if( Vterm>Vcapasum) ssx=1;
      |             else  ssx=0;
      |         }
      | 
      |         x_keep[k]=Ad[ssx]*Vcap[k];  //+Bd1[ssx]*I;    Bd1=0 avec backward Euler                                                          // note: with BE Bd1=0
      |         Vhist+=(C[ssx]*x_keep[k]);    //V_hist =V_hist + C(k)*state_tmp(k);  % compute Thevenin voltage
      | 
      |         Zmmc+=Z[ssx];  // Z = sum(C'.*Bd2 + D);  Y=inv(Z)
      | 
      |         Bd2keep[k]=Bd2[ssx];
      |         gate[k]=ssx;
      |         *(Vcap_out+k)=Vcap[k];
      |         }
      | 
      | 
      |     Ymmc=1/Zmmc;    // admittance= inverse of the sum of cell impedance
      |     Ihist=Vhist*Ymmc;  // history source
      | 
      |     state_keep[0]=Vhist;
      | 
      |     Y=Ymmc;
      | 
      |     state_keep[1]=Ymmc;
      | 
      |     Immc=0.0-I;
      | 
      | }
      CodegenInitializeConditionsCode=|
      | for (int i=0; i<nbc ;i++){
      |     x_keep[i]=0;
      |     Bd2keep[i]*0;
      |     Vc_state[i]=0;
      |     gate[i]=0;
      |     Vcap[i]=0;
      |     }
      |     
      |     state=0;
      |     state_keep[0]=0;
      |     state_keep[1]=0;
  Controlled Current Source : fl_lib/Electrical/Electrical Sources/Controlled Current Source
  Divide : Product  Inputs=/
  Gain -1 (SSN correct polarity of injection)1 : Gain
  PS-Simulink Converter2 : nesl_utility/PS-Simulink Converter  PhysicalDomain=network_engine_domain  SubClassName=ps_output  LeftPortType=input  RightPortType=output  PseudoPeriodic=off  Frequencies=[]  VectorFormat=inherit  Unit=inherit  AffineConversion=off
  Saturation : Saturate  UpperLimit=1e9  LowerLimit=0
  Simulink-PS Converter : nesl_utility/Simulink-PS Converter  PhysicalDomain=network_engine_domain  SubClassName=ps_input  LeftPortType=input  RightPortType=output  PseudoPeriodic=off  Frequencies=[]  NoiseDistribution=none  NoiseParameters=[]  Unit=1  AffineConversion=off  FilteringAndDerivatives=provide  SimscapeFilterOrder=1  InputFilterTimeConstant=0.001  UdotUserProvided=0
  Simulink-PS Converter1 : nesl_utility/Simulink-PS Converter  PhysicalDomain=network_engine_domain  SubClassName=ps_input  LeftPortType=input  RightPortType=output  PseudoPeriodic=off  Frequencies=[]  NoiseDistribution=none  NoiseParameters=[]  Unit=1  AffineConversion=off  FilteringAndDerivatives=provide  SimscapeFilterOrder=1  InputFilterTimeConstant=0.001  UdotUserProvided=0
  Subsystem : Subsystem  mask(MMC pulsing){nbc=nbc}
      mask prompts: nbc "Number of Cells"
      mask init:
      | igbtorder=[];
      | for i=1:nbc
      |     igbtorder=[igbtorder i i+nbc];
      | end
      | igbtorder;
  Unit Delay : UnitDelay  SampleTime=Ts  HasFrameUpgradeWarning=on
  Variable Resistor : fl_lib/Electrical/Electrical Elements/Variable Resistor  Rmin=1e-8 Ohm  thermalEnable=false  thermal_mass=1 J/K  i_specify=off  i_priority=None  i=0 A  i_nominal_specify=off  i_nominal_value=1  i_nominal_unit=A  v_specify=off  v_priority=None  v=0 V  v_nominal_specify=off  v_nominal_value=1  v_nominal_unit=V  T_specify=off  T_priority=None  T=300 K  T_nominal_specify=off  T_nominal_value=1  T_nominal_unit=K
  Voltage Sensor : fl_lib/Electrical/Electrical Sensors/Voltage Sensor
  +V : PMIOPort  Side=Left
  -V : PMIOPort  Port=2  Side=Left
  iv : Outport  VectorParamsAs1DForOutWhenUnconnected=off
  Vcap : Outport  Port=2  VectorParamsAs1DForOutWhenUnconnected=off
  wires:
  Saturation/1 -> Divide/1
  Divide/1 -> Simulink-PS Converter/1
  Gain -1 (SSN correct polarity of injection)1/1 -> Simulink-PS Converter1/1
  [Vnode_ssc] -> Unit Delay/1
  PS-Simulink Converter2/1 -> [Vnode_ssc]
  deblock/1 -> Subsystem/2(en)
  Subsystem/2(outN) -> C Function1/2
  Pulse/1 -> Subsystem/1(gup)
  Subsystem/1(out) -> C Function1/1
  Bus Creator5/1 -> iv/1
  Unit Delay/1 -> C Function1/3, Bus Creator5/2  "Vc"
  C Function1/1 -> Saturation/1
  C Function1/2 -> Gain -1 (SSN correct polarity of injection)1/1
  C Function1/3 -> Vcap/1
  C Function1/4 -> Bus Creator5/1  "Iin"
  connections:
  Controlled Current Source/RConn1 -- Simulink-PS Converter1/RConn1
  PS-Simulink Converter2/LConn1 -- Voltage Sensor/RConn1
  Variable Resistor/RConn1 -- +V/RConn1 -- Controlled Current Source/LConn1 -- Voltage Sensor/LConn1
  Variable Resistor/LConn2 -- -V/RConn1 -- Controlled Current Source/RConn2 -- Voltage Sensor/RConn2
  Simulink-PS Converter/RConn1 -- Variable Resistor/LConn1

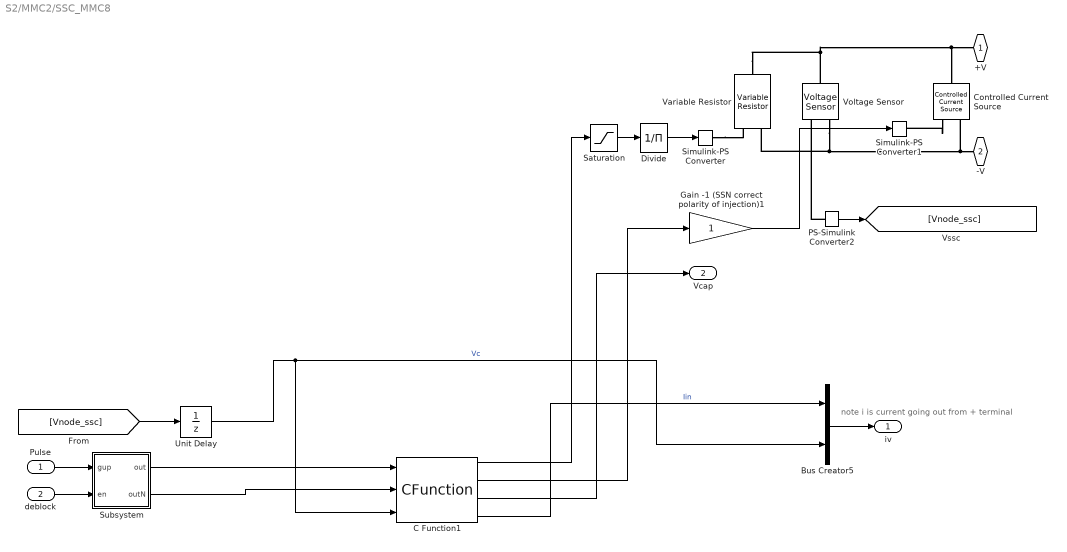
== system S2/MMC2/SSC_MMC8 ==
  note: note i is current going out from + terminal
  Pulse : Inport
  deblock : Inport  Port=2
  Bus Creator5 : BusCreator  Inputs=2
  C Function1 : CFunction  OutputCode=|  StartCode=state = initialValue;  InitializeConditionsCode=|  CodegenOutputCode=|  CodegenStartCode=state = initialValue;  CodegenInitializeConditionsCode=|  SampleTime=SampleTime  CustomCodeSettingLocation=ModelConfigurationParameters  initialValue=0  Ad=Ad  Bd2=Bd2  C=C  nbc=nbc  Z=Z  SampleTime=-1
      OutputCode=|
      | {
      | 
      | int ssx;
      | double Vcapasum, Ymmc, Zmmc, Vhist, Vterm;
      | double I;
      | 
      | Vcapasum=0;
      | I=(Vnodal- state_keep[0])* state_keep[1];  
      | 
      |     for (int k=0;k<nbc;k++){ //  % scan of cells to complete state-space iteration
      |         Vcap[k]=x_keep[k]+Bd2keep[k]*I;
      |         if (*(g_lower+k)<0.5) Vcapasum+=Vcap[k]; // sum all non-shorted capacitor voltages
      |     }
      | 
      | 
      |     Vhist=0;  // reset Vhist
      |     Zmmc=0;  // reset
      |     Vterm=  Vnodal;
      | 
      | 
      |     // we calculate the cells conduction states from the gate values.
      |     for (int k=0;k<nbc;k++){
      |         // ss=2-> lower IGBT/diode ON
      |         // ss=1-> upper IGBT/diode ON  //attention!!!!
      |         // ss=0-> hi-Z
      |         ssx=(int)gate[k];
      |         if (*(g_lower+k)>0.5) ssx=2;
      |         else if (*(g_upper+k)>0.5) ssx=1;
      |         else {
      |             if  (Vterm<0)  ssx=2;
      |             else if( Vterm>Vcapasum) ssx=1;
      |             else  ssx=0;
      |         }
      | 
      |         x_keep[k]=Ad[ssx]*Vcap[k];  //+Bd1[ssx]*I;    Bd1=0 avec backward Euler                                                          // note: with BE Bd1=0
      |         Vhist+=(C[ssx]*x_keep[k]);    //V_hist =V_hist + C(k)*state_tmp(k);  % compute Thevenin voltage
      | 
      |         Zmmc+=Z[ssx];  // Z = sum(C'.*Bd2 + D);  Y=inv(Z)
      | 
      |         Bd2keep[k]=Bd2[ssx];
      |         gate[k]=ssx;
      |         *(Vcap_out+k)=Vcap[k];
      |         }
      | 
      | 
      |     Ymmc=1/Zmmc;    // admittance= inverse of the sum of cell impedance
      |     Ihist=Vhist*Ymmc;  // history source
      | 
      |     state_keep[0]=Vhist;
      | 
      |     Y=Ymmc;
      | 
      |     state_keep[1]=Ymmc;
      | 
      |     Immc=0.0-I;
      | 
      | }
      InitializeConditionsCode=|
      | for (int i=0; i<nbc ;i++){
      |     x_keep[i]=0;
      |     Bd2keep[i]*0;
      |     Vc_state[i]=0;
      |     gate[i]=0;
      |     Vcap[i]=0;
      |     }
      |     
      |     state=0;
      |     state_keep[0]=0;
      |     state_keep[1]=0;
      CodegenOutputCode=|
      | {
      | 
      | int ssx;
      | double Vcapasum, Ymmc, Zmmc, Vhist, Vterm;
      | double I;
      | 
      | Vcapasum=0;
      | I=(Vnodal- state_keep[0])* state_keep[1];  
      | 
      |     for (int k=0;k<nbc;k++){ //  % scan of cells to complete state-space iteration
      |         Vcap[k]=x_keep[k]+Bd2keep[k]*I;
      |         if (*(g_lower+k)<0.5) Vcapasum+=Vcap[k]; // sum all non-shorted capacitor voltages
      |     }
      | 
      | 
      |     Vhist=0;  // reset Vhist
      |     Zmmc=0;  // reset
      |     Vterm=  Vnodal;
      | 
      | 
      |     // we calculate the cells conduction states from the gate values.
      |     for (int k=0;k<nbc;k++){
      |         // ss=2-> lower IGBT/diode ON
      |         // ss=1-> upper IGBT/diode ON  //attention!!!!
      |         // ss=0-> hi-Z
      |         ssx=(int)gate[k];
      |         if (*(g_lower+k)>0.5) ssx=2;
      |         else if (*(g_upper+k)>0.5) ssx=1;
      |         else {
      |             if  (Vterm<0)  ssx=2;
      |             else if( Vterm>Vcapasum) ssx=1;
      |             else  ssx=0;
      |         }
      | 
      |         x_keep[k]=Ad[ssx]*Vcap[k];  //+Bd1[ssx]*I;    Bd1=0 avec backward Euler                                                          // note: with BE Bd1=0
      |         Vhist+=(C[ssx]*x_keep[k]);    //V_hist =V_hist + C(k)*state_tmp(k);  % compute Thevenin voltage
      | 
      |         Zmmc+=Z[ssx];  // Z = sum(C'.*Bd2 + D);  Y=inv(Z)
      | 
      |         Bd2keep[k]=Bd2[ssx];
      |         gate[k]=ssx;
      |         *(Vcap_out+k)=Vcap[k];
      |         }
      | 
      | 
      |     Ymmc=1/Zmmc;    // admittance= inverse of the sum of cell impedance
      |     Ihist=Vhist*Ymmc;  // history source
      | 
      |     state_keep[0]=Vhist;
      | 
      |     Y=Ymmc;
      | 
      |     state_keep[1]=Ymmc;
      | 
      |     Immc=0.0-I;
      | 
      | }
      CodegenInitializeConditionsCode=|
      | for (int i=0; i<nbc ;i++){
      |     x_keep[i]=0;
      |     Bd2keep[i]*0;
      |     Vc_state[i]=0;
      |     gate[i]=0;
      |     Vcap[i]=0;
      |     }
      |     
      |     state=0;
      |     state_keep[0]=0;
      |     state_keep[1]=0;
  Controlled Current Source : fl_lib/Electrical/Electrical Sources/Controlled Current Source
  Divide : Product  Inputs=/
  Gain -1 (SSN correct polarity of injection)1 : Gain
  PS-Simulink Converter2 : nesl_utility/PS-Simulink Converter  PhysicalDomain=network_engine_domain  SubClassName=ps_output  LeftPortType=input  RightPortType=output  PseudoPeriodic=off  Frequencies=[]  VectorFormat=inherit  Unit=inherit  AffineConversion=off
  Saturation : Saturate  UpperLimit=1e9  LowerLimit=0
  Simulink-PS Converter : nesl_utility/Simulink-PS Converter  PhysicalDomain=network_engine_domain  SubClassName=ps_input  LeftPortType=input  RightPortType=output  PseudoPeriodic=off  Frequencies=[]  NoiseDistribution=none  NoiseParameters=[]  Unit=1  AffineConversion=off  FilteringAndDerivatives=provide  SimscapeFilterOrder=1  InputFilterTimeConstant=0.001  UdotUserProvided=0
  Simulink-PS Converter1 : nesl_utility/Simulink-PS Converter  PhysicalDomain=network_engine_domain  SubClassName=ps_input  LeftPortType=input  RightPortType=output  PseudoPeriodic=off  Frequencies=[]  NoiseDistribution=none  NoiseParameters=[]  Unit=1  AffineConversion=off  FilteringAndDerivatives=provide  SimscapeFilterOrder=1  InputFilterTimeConstant=0.001  UdotUserProvided=0
  Subsystem : Subsystem  mask(MMC pulsing){nbc=nbc}
      mask prompts: nbc "Number of Cells"
      mask init:
      | igbtorder=[];
      | for i=1:nbc
      |     igbtorder=[igbtorder i i+nbc];
      | end
      | igbtorder;
  Unit Delay : UnitDelay  SampleTime=Ts  HasFrameUpgradeWarning=on
  Variable Resistor : fl_lib/Electrical/Electrical Elements/Variable Resistor  Rmin=1e-8 Ohm  thermalEnable=false  thermal_mass=1 J/K  i_specify=off  i_priority=None  i=0 A  i_nominal_specify=off  i_nominal_value=1  i_nominal_unit=A  v_specify=off  v_priority=None  v=0 V  v_nominal_specify=off  v_nominal_value=1  v_nominal_unit=V  T_specify=off  T_priority=None  T=300 K  T_nominal_specify=off  T_nominal_value=1  T_nominal_unit=K
  Voltage Sensor : fl_lib/Electrical/Electrical Sensors/Voltage Sensor
  +V : PMIOPort  Side=Left
  -V : PMIOPort  Port=2  Side=Left
  iv : Outport  VectorParamsAs1DForOutWhenUnconnected=off
  Vcap : Outport  Port=2  VectorParamsAs1DForOutWhenUnconnected=off
  wires:
  Saturation/1 -> Divide/1
  Divide/1 -> Simulink-PS Converter/1
  Gain -1 (SSN correct polarity of injection)1/1 -> Simulink-PS Converter1/1
  [Vnode_ssc] -> Unit Delay/1
  PS-Simulink Converter2/1 -> [Vnode_ssc]
  deblock/1 -> Subsystem/2(en)
  Subsystem/2(outN) -> C Function1/2
  Pulse/1 -> Subsystem/1(gup)
  Subsystem/1(out) -> C Function1/1
  Bus Creator5/1 -> iv/1
  Unit Delay/1 -> C Function1/3, Bus Creator5/2  "Vc"
  C Function1/1 -> Saturation/1
  C Function1/2 -> Gain -1 (SSN correct polarity of injection)1/1
  C Function1/3 -> Vcap/1
  C Function1/4 -> Bus Creator5/1  "Iin"
  connections:
  Controlled Current Source/RConn1 -- Simulink-PS Converter1/RConn1
  PS-Simulink Converter2/LConn1 -- Voltage Sensor/RConn1
  Variable Resistor/RConn1 -- +V/RConn1 -- Controlled Current Source/LConn1 -- Voltage Sensor/LConn1
  Variable Resistor/LConn2 -- -V/RConn1 -- Controlled Current Source/RConn2 -- Voltage Sensor/RConn2
  Simulink-PS Converter/RConn1 -- Variable Resistor/LConn1

== system S2/Half-DPL1ph1/dplmodel/derlay ==
  In1 : Inport
  Add : Sum
  Delay1 : Delay  DelayLength=delay(1)
  Gain : Gain  Gain=remd
  Gain1 : Gain  Gain=1-remd
  Unit Delay1 : UnitDelay  SampleTime=Ts  HasFrameUpgradeWarning=on
  Out1 : Outport
  wires:
  Delay1/1 -> Unit Delay1/1, Gain1/1
  Add/1 -> Out1/1
  Unit Delay1/1 -> Gain/1
  Gain1/1 -> Add/2
  Gain/1 -> Add/1
  In1/1 -> Delay1/1

== system S2/Half-DPL1ph2/dplmodel/derlay ==
  In1 : Inport
  Add : Sum
  Delay1 : Delay  DelayLength=delay(1)
  Gain : Gain  Gain=remd
  Gain1 : Gain  Gain=1-remd
  Unit Delay1 : UnitDelay  SampleTime=Ts  HasFrameUpgradeWarning=on
  Out1 : Outport
  wires:
  In1/1 -> Delay1/1
  Gain/1 -> Add/1
  Gain1/1 -> Add/2
  Unit Delay1/1 -> Gain/1
  Add/1 -> Out1/1
  Delay1/1 -> Gain1/1, Unit Delay1/1

== system S2/MMC2/ Switch Identifier1/inv1 ==
  gate : Inport
  Constant1 : Constant
  Sum3 : Sum  Inputs=-+
  Out1 : Outport
  wires:
  Sum3/1 -> Out1/1
  gate/1 -> Sum3/1
  Constant1/1 -> Sum3/2

== system S2/MMC2/ Switch Identifier2/inv1 ==
  gate : Inport
  Constant1 : Constant
  Sum3 : Sum  Inputs=-+
  Out1 : Outport
  wires:
  Sum3/1 -> Out1/1
  gate/1 -> Sum3/1
  Constant1/1 -> Sum3/2

== system S2/MMC2/ Switch Identifier3/inv1 ==
  gate : Inport
  Constant1 : Constant
  Sum3 : Sum  Inputs=-+
  Out1 : Outport
  wires:
  Sum3/1 -> Out1/1
  gate/1 -> Sum3/1
  Constant1/1 -> Sum3/2

== system S2/MMC2/SSC_MMC1/Subsystem ==
  gup : Inport
  en : Inport  Port=2
  Compare To Constant : simulink/Logic and Bit Operations/Compare To Constant  relop=>=  const=0.5  OutDataTypeStr=boolean
  Data Type Conversion : DataTypeConversion  OutDataTypeStr=double  SaturateOnIntegerOverflow=off  RndMeth=Floor
  Data Type Conversion1 : DataTypeConversion  OutDataTypeStr=double  SaturateOnIntegerOverflow=off  RndMeth=Floor
  Divide : Product
  Divide1 : Product
  Logical Operator1 : Logic  Operator=NOT  Inputs=1  AllPortsSameDT=off  OutDataTypeStr=boolean
  out : Outport  VectorParamsAs1DForOutWhenUnconnected=off
  outN : Outport  Port=2  VectorParamsAs1DForOutWhenUnconnected=off
  wires:
  Divide1/1 -> outN/1
  Divide/1 -> out/1
  Data Type Conversion1/1 -> Divide/2
  Data Type Conversion/1 -> Divide1/1
  en/1 -> Divide1/2, Divide/1
  Compare To Constant/1 -> Logical Operator1/1, Data Type Conversion1/1
  Logical Operator1/1 -> Data Type Conversion/1
  gup/1 -> Compare To Constant/1

== system S2/MMC2/SSC_MMC2/Subsystem ==
  gup : Inport
  en : Inport  Port=2
  Compare To Constant : simulink/Logic and Bit Operations/Compare To Constant  relop=>=  const=0.5  OutDataTypeStr=boolean
  Data Type Conversion : DataTypeConversion  OutDataTypeStr=double  SaturateOnIntegerOverflow=off  RndMeth=Floor
  Data Type Conversion1 : DataTypeConversion  OutDataTypeStr=double  SaturateOnIntegerOverflow=off  RndMeth=Floor
  Divide : Product
  Divide1 : Product
  Logical Operator1 : Logic  Operator=NOT  Inputs=1  AllPortsSameDT=off  OutDataTypeStr=boolean
  out : Outport  VectorParamsAs1DForOutWhenUnconnected=off
  outN : Outport  Port=2  VectorParamsAs1DForOutWhenUnconnected=off
  wires:
  gup/1 -> Compare To Constant/1
  Logical Operator1/1 -> Data Type Conversion/1
  Compare To Constant/1 -> Data Type Conversion1/1, Logical Operator1/1
  en/1 -> Divide/1, Divide1/2
  Data Type Conversion/1 -> Divide1/1
  Data Type Conversion1/1 -> Divide/2
  Divide/1 -> out/1
  Divide1/1 -> outN/1

== system S2/MMC2/SSC_MMC3/Subsystem ==
  gup : Inport
  en : Inport  Port=2
  Compare To Constant : simulink/Logic and Bit Operations/Compare To Constant  relop=>=  const=0.5  OutDataTypeStr=boolean
  Data Type Conversion : DataTypeConversion  OutDataTypeStr=double  SaturateOnIntegerOverflow=off  RndMeth=Floor
  Data Type Conversion1 : DataTypeConversion  OutDataTypeStr=double  SaturateOnIntegerOverflow=off  RndMeth=Floor
  Divide : Product
  Divide1 : Product
  Logical Operator1 : Logic  Operator=NOT  Inputs=1  AllPortsSameDT=off  OutDataTypeStr=boolean
  out : Outport  VectorParamsAs1DForOutWhenUnconnected=off
  outN : Outport  Port=2  VectorParamsAs1DForOutWhenUnconnected=off
  wires:
  Divide1/1 -> outN/1
  Divide/1 -> out/1
  Data Type Conversion1/1 -> Divide/2
  Data Type Conversion/1 -> Divide1/1
  en/1 -> Divide1/2, Divide/1
  Compare To Constant/1 -> Logical Operator1/1, Data Type Conversion1/1
  Logical Operator1/1 -> Data Type Conversion/1
  gup/1 -> Compare To Constant/1

== system S2/MMC2/SSC_MMC4/Subsystem ==
  gup : Inport
  en : Inport  Port=2
  Compare To Constant : simulink/Logic and Bit Operations/Compare To Constant  relop=>=  const=0.5  OutDataTypeStr=boolean
  Data Type Conversion : DataTypeConversion  OutDataTypeStr=double  SaturateOnIntegerOverflow=off  RndMeth=Floor
  Data Type Conversion1 : DataTypeConversion  OutDataTypeStr=double  SaturateOnIntegerOverflow=off  RndMeth=Floor
  Divide : Product
  Divide1 : Product
  Logical Operator1 : Logic  Operator=NOT  Inputs=1  AllPortsSameDT=off  OutDataTypeStr=boolean
  out : Outport  VectorParamsAs1DForOutWhenUnconnected=off
  outN : Outport  Port=2  VectorParamsAs1DForOutWhenUnconnected=off
  wires:
  Divide1/1 -> outN/1
  Divide/1 -> out/1
  Data Type Conversion1/1 -> Divide/2
  Data Type Conversion/1 -> Divide1/1
  en/1 -> Divide1/2, Divide/1
  Compare To Constant/1 -> Logical Operator1/1, Data Type Conversion1/1
  Logical Operator1/1 -> Data Type Conversion/1
  gup/1 -> Compare To Constant/1

== system S2/MMC2/SSC_MMC5/Subsystem ==
  gup : Inport
  en : Inport  Port=2
  Compare To Constant : simulink/Logic and Bit Operations/Compare To Constant  relop=>=  const=0.5  OutDataTypeStr=boolean
  Data Type Conversion : DataTypeConversion  OutDataTypeStr=double  SaturateOnIntegerOverflow=off  RndMeth=Floor
  Data Type Conversion1 : DataTypeConversion  OutDataTypeStr=double  SaturateOnIntegerOverflow=off  RndMeth=Floor
  Divide : Product
  Divide1 : Product
  Logical Operator1 : Logic  Operator=NOT  Inputs=1  AllPortsSameDT=off  OutDataTypeStr=boolean
  out : Outport  VectorParamsAs1DForOutWhenUnconnected=off
  outN : Outport  Port=2  VectorParamsAs1DForOutWhenUnconnected=off
  wires:
  gup/1 -> Compare To Constant/1
  Logical Operator1/1 -> Data Type Conversion/1
  Compare To Constant/1 -> Data Type Conversion1/1, Logical Operator1/1
  en/1 -> Divide/1, Divide1/2
  Data Type Conversion/1 -> Divide1/1
  Data Type Conversion1/1 -> Divide/2
  Divide/1 -> out/1
  Divide1/1 -> outN/1

== system S2/MMC2/SSC_MMC8/Subsystem ==
  gup : Inport
  en : Inport  Port=2
  Compare To Constant : simulink/Logic and Bit Operations/Compare To Constant  relop=>=  const=0.5  OutDataTypeStr=boolean
  Data Type Conversion : DataTypeConversion  OutDataTypeStr=double  SaturateOnIntegerOverflow=off  RndMeth=Floor
  Data Type Conversion1 : DataTypeConversion  OutDataTypeStr=double  SaturateOnIntegerOverflow=off  RndMeth=Floor
  Divide : Product
  Divide1 : Product
  Logical Operator1 : Logic  Operator=NOT  Inputs=1  AllPortsSameDT=off  OutDataTypeStr=boolean
  out : Outport  VectorParamsAs1DForOutWhenUnconnected=off
  outN : Outport  Port=2  VectorParamsAs1DForOutWhenUnconnected=off
  wires:
  gup/1 -> Compare To Constant/1
  Logical Operator1/1 -> Data Type Conversion/1
  Compare To Constant/1 -> Data Type Conversion1/1, Logical Operator1/1
  en/1 -> Divide/1, Divide1/2
  Data Type Conversion/1 -> Divide1/1
  Data Type Conversion1/1 -> Divide/2
  Divide/1 -> out/1
  Divide1/1 -> outN/1
